simulink model "lab02_3"  (R2022a)
settings: Solver=ode45  StartTime=0.0  StopTime=3  MaxStep=0.001  RelTol=1e-3
values from neighbouring files (symbols this model uses):
  a = 2.5    [part3_plot.m]
settings Model: Creator=yg  LastModifiedBy=zhong
settings DebuggingCC: UnconnectedInputMsg=warning  UnconnectedOutputMsg=warning  UnconnectedLineMsg=warning
settings RTWCC: DLArmComputeVersion=19.05

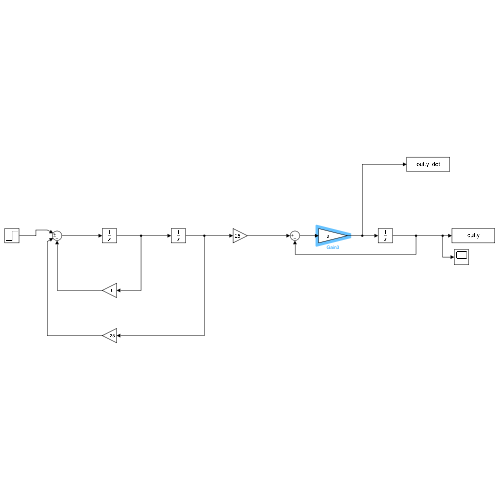
[thumbnail: Simulink's stored preview of the top-level diagram]
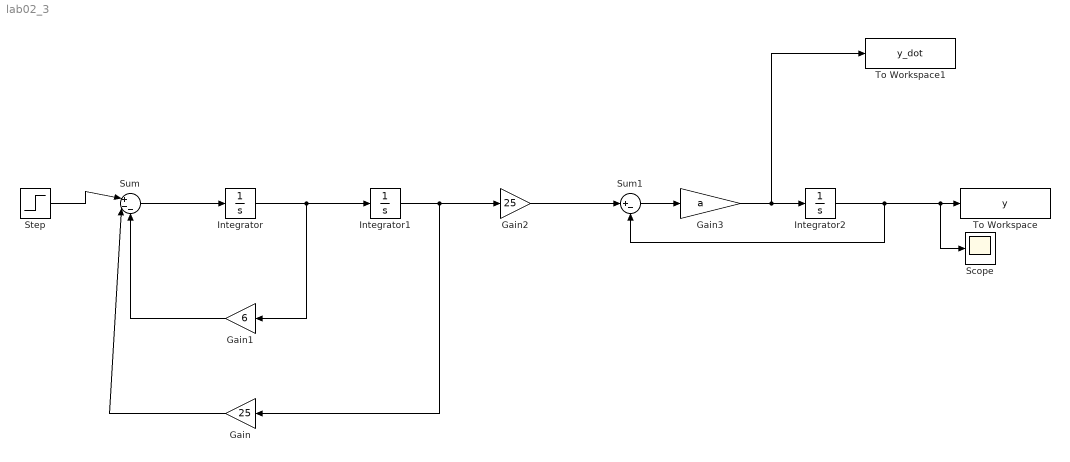
== system lab02_3 ==
  Gain : Gain  Gain=25
  Gain1 : Gain  Gain=6
  Gain2 : Gain  Gain=25
  Gain3 : Gain  Gain=a
  Integrator : Integrator
  Integrator1 : Integrator
  Integrator2 : Integrator
  Scope : Scope
  Step : Step  Time=0  SampleTime=0
  Sum : Sum  Inputs=|+--
  Sum1 : Sum  Inputs=|+-
  To Workspace : ToWorkspace  VariableName=y  SampleTime=-1
  To Workspace1 : ToWorkspace  VariableName=y_dot  SampleTime=-1
  wires:
  Sum/1 -> Integrator/1
  Integrator/1 -> Gain1/1, Integrator1/1
  Gain1/1 -> Sum/3
  Integrator1/1 -> Gain/1, Gain2/1
  Gain/1 -> Sum/2
  Step/1 -> Sum/1
  Gain2/1 -> Sum1/1
  Sum1/1 -> Gain3/1
  Integrator2/1 -> Scope/1, To Workspace/1, Sum1/2
  Gain3/1 -> Integrator2/1, To Workspace1/1
